simulink model "s11_16"  (Simulink 6.6)
settings: Solver=ode45  StartTime=0.0  StopTime=T  MaxStep=0.01  RelTol=1e-3
values from neighbouring files (symbols this model uses):
  theta_0 = -pi/2    (= -1.57079632679)    [i11_16.m]
  x_0 = -1    [i11_16.m]
  y_0 = -2    [i11_16.m]
undefined symbols (not defined in the file or in its folder): cart_reg
settings Model: Creator=marilena  LastModifiedBy=luigivillani  ExtModeAutoUpdateStatusClock=off
settings OptimizationCC: InitFltsAndDblsToZero=off
settings HardwareCC: TargetHWDeviceType=32-bit Generic

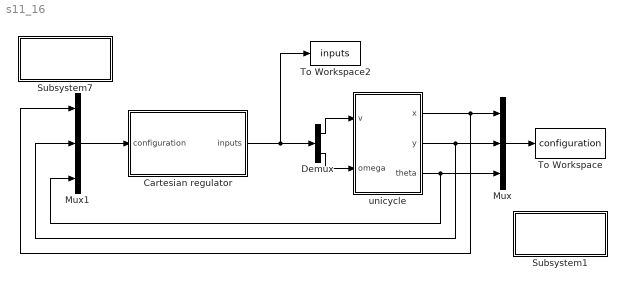
== system s11_16 ==
  Cartesian regulator : Subsystem
  Demux : Demux  Outputs=2
  Mux : Mux  Inputs=3
  Mux1 : Mux  Inputs=3
  Subsystem1 : Subsystem
      settings: OpenFcn=p11_16
      mask Display: disp('plot')
  Subsystem7 : Subsystem
      settings: OpenFcn=i11_16
      mask Display: disp('variables\n initialization')
  To Workspace : ToWorkspace  VariableName=configuration  SampleTime=-1  SaveFormat=Structure With Time
  To Workspace2 : ToWorkspace  VariableName=inputs  SampleTime=-1  SaveFormat=Structure With Time
  unicycle : Subsystem
  wires:
  Mux/1 -> To Workspace/1
  unicycle/3(theta) -> Mux/3, Mux1/3
  unicycle/1(x) -> Mux/1, Mux1/1
  Mux1/1 -> Cartesian regulator/1(configuration)
  Cartesian regulator/1(inputs) -> Demux/1, To Workspace2/1
  unicycle/2(y) -> Mux/2, Mux1/2
  Demux/1 -> unicycle/1(v)
  Demux/2 -> unicycle/2(omega)

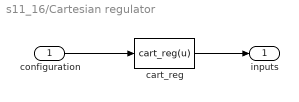
== system s11_16/Cartesian regulator ==
  configuration : Inport
  cart_reg : MATLABFcn  Tag={'prova'}  Description=cartesian regulator  MATLABFcn=cart_reg(u)  Output1D=off
  inputs : Outport
  wires:
  configuration/1 -> cart_reg/1
  cart_reg/1 -> inputs/1

== system s11_16/Subsystem1 ==

== system s11_16/Subsystem7 ==

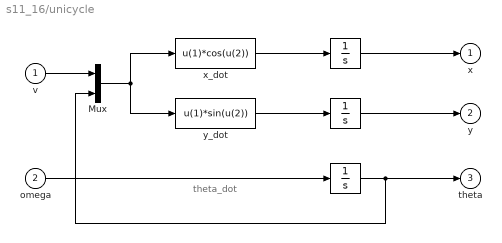
== system s11_16/unicycle ==
  note: theta_dot
  v : Inport  OutDataType=fixdt(1,16,0)  OutScaling=[]
  omega : Inport  Port=2  OutDataType=fixdt(1,16,0)  OutScaling=[]
  " " : Integrator  InitialCondition=theta_0
  "   " : Integrator  InitialCondition=x_0
  "    " : Integrator  InitialCondition=y_0
  Mux : Mux  Inputs=2
  x_dot : Fcn  Expr=u(1)*cos(u(2))
  y_dot : Fcn  Expr=u(1)*sin(u(2))
  x : Outport  OutDataType=fixdt(1,16,0)  OutScaling=[]
  y : Outport  Port=2  OutDataType=fixdt(1,16,0)  OutScaling=[]
  theta : Outport  Port=3  OutDataType=fixdt(1,16,0)  OutScaling=[]
  wires:
  v/1 -> Mux/1
  omega/1 -> " "/1
  x_dot/1 -> "   "/1
  y_dot/1 -> "    "/1
  " "/1 -> Mux/2, theta/1
  Mux/1 -> x_dot/1, y_dot/1
  "   "/1 -> x/1
  "    "/1 -> y/1
